simulink library "TYPEBP_MASTER_tmp"  (Simulink 8.6)
settings: Solver=ode45  StartTime=0.0  StopTime=10.0  RelTol=1e-3
undefined symbols (not defined in the file): TYPEC, TYPEC_MASTER
libraries: cdsEpicsOut x112, cdsFilt x79, cdsTP x59, cdsFiltCtrl x36, VIS_LIB x20, cdsEpicsIn x18, cdsMuxMatrix x14, STATE_BIO_MASTER x12, cdsEpicsBinIn x8, cdsFunctionCall x4, lockin x4, cdsEpicsStringIn x2
(part 12 of 13)

== system TYPEBP_MASTER_tmp/TYPEBPMASTER_TEST/SF/TEST ==
  GAS : cdsFilt/Subsystem  Tag=cdsFilt  Description=|
      | Purpose:                                                                                                                                                                                                                                  
      | Standard CDS IIR filter module.                                                                                                                                                                                                           
      |                                                                                                                                                                                                                                           
      | Operation:                                                                                                                                                                                                                                
      | Consists of 10 second order section IIR filters, plus a ramped gain stage. In FE code, also provides pre-defined test points and excitation channel inputs. The filter coefficients are defined in the LIGO system using the 'foton' tool.
      |                                                                                                                                                                                                                                           
      | Usage:                                                                                                                                                                                                                                    
      | Name the part with the desired filter module name.
      settings: AttributesFormatString=%<Tag>
  Ground1 : Ground
  Ground7 : Ground
  STATUS : cdsEpicsBinIn/Subsystem  Tag=cdsEpicsBinIn  Description=|
      | Purpose:                                                                            
      | Create an EPICS binary (0 or 1) input channel to the FE realtime controls.          
      |                                                                                     
      | Operation:                                                                          
      | Outputs value from an EPICS ai record. Value is binary input (bi Epics record type).
      |                                                                                     
      | Usage:                                                                              
      | Name the part with the desired EPICS channel name.
      settings: AttributesFormatString=%<Tag>
  F0_Out : Outport
  wires:
  GAS/1 -> F0_Out/1
  Ground1/1 -> GAS/1
  Ground7/1 -> STATUS/1

== system TYPEBP_MASTER_tmp/TYPEBPMASTER_TEST/TM/ADD ==
  ISC_L_In : Inport
  ISC_P_In : Inport  Port=2
  ISC_Y_In : Inport  Port=3
  TEST_L_In : Inport  Port=4
  TEST_P_In : Inport  Port=5
  TEST_Y_In : Inport  Port=6
  DAMP_L_In : Inport  Port=7
  DAMP_P_In : Inport  Port=8
  DAMP_Y_In : Inport  Port=9
  Ground{1..6} (6 alike) : Ground
  L : cdsFiltCtrl/IIR FM with control  Tag=cdsFiltCtrl  Description=|
      | cdsFiltCntrl is the standard IIR filter module (exactly the same as cdsFilt) but with added control data output 'Ctrl'. Filter module digital signal output appears on the first output, which is called 'Val'. 'Ctrl' output has a bit pattern encoding the state of filter's on/off switches (FM1 through FM10). The bit values are:
      |                                                                                                                                                                                                                                                                                                                                       
      | module 	hex	dec                                                                                                                                                                                                                                                                                                                       
      | -----------------------                                                                                                                                                                                                                                                                                                               
      | FM1	0x20                    32                                                                                                                                                                                                                                                                                                        
      | FM2	0x80                     128                                                                                                                                                                                                                                                                                                      
      | FM3	0x200                   512                                                                                                                                                                                                                                                                                                       
      | FM4	0x800                   2048                                                                                                                                                                                                                                                                                                      
      | FM5	0x2000                 8192                                                                                                                                                                                                                                                                                                       
      | FM6	0x8000                 32768                                                                                                                                                                                                                                                                                                      
      | FM7	0x20000                131072                                                                                                                                                                                                                                                                                                     
      | FM8	0x80000                 524288                                                                                                                                                                                                                                                                                                    
      | FM9	0x200000               2097152                                                                                                                                                                                                                                                                                                    
      | FM10	0x800000               8388608                                                                                                                                                                                                                                                                                                   
      |                                                                                                                                                                                                                                                                                                                                       
      | This bit data can be used to drive some other switches or it can be output using a binary I/O module.
      settings: AttributesFormatString=%<Tag>
  P : cdsFiltCtrl/IIR FM with control  Tag=cdsFiltCtrl  Description=|
      | cdsFiltCntrl is the standard IIR filter module (exactly the same as cdsFilt) but with added control data output 'Ctrl'. Filter module digital signal output appears on the first output, which is called 'Val'. 'Ctrl' output has a bit pattern encoding the state of filter's on/off switches (FM1 through FM10). The bit values are:
      |                                                                                                                                                                                                                                                                                                                                       
      | module 	hex	dec                                                                                                                                                                                                                                                                                                                       
      | -----------------------                                                                                                                                                                                                                                                                                                               
      | FM1	0x20                    32                                                                                                                                                                                                                                                                                                        
      | FM2	0x80                     128                                                                                                                                                                                                                                                                                                      
      | FM3	0x200                   512                                                                                                                                                                                                                                                                                                       
      | FM4	0x800                   2048                                                                                                                                                                                                                                                                                                      
      | FM5	0x2000                 8192                                                                                                                                                                                                                                                                                                       
      | FM6	0x8000                 32768                                                                                                                                                                                                                                                                                                      
      | FM7	0x20000                131072                                                                                                                                                                                                                                                                                                     
      | FM8	0x80000                 524288                                                                                                                                                                                                                                                                                                    
      | FM9	0x200000               2097152                                                                                                                                                                                                                                                                                                    
      | FM10	0x800000               8388608                                                                                                                                                                                                                                                                                                   
      |                                                                                                                                                                                                                                                                                                                                       
      | This bit data can be used to drive some other switches or it can be output using a binary I/O module.
      settings: AttributesFormatString=%<Tag>
  Sum : Sum  Inputs=+++
  Sum3 : Sum  Inputs=+++
  Sum4 : Sum  Inputs=+++
  Terminator1 : Terminator
  Terminator2 : Terminator
  Terminator3 : Terminator
  Y : cdsFiltCtrl/IIR FM with control  Tag=cdsFiltCtrl  Description=|
      | cdsFiltCntrl is the standard IIR filter module (exactly the same as cdsFilt) but with added control data output 'Ctrl'. Filter module digital signal output appears on the first output, which is called 'Val'. 'Ctrl' output has a bit pattern encoding the state of filter's on/off switches (FM1 through FM10). The bit values are:
      |                                                                                                                                                                                                                                                                                                                                       
      | module 	hex	dec                                                                                                                                                                                                                                                                                                                       
      | -----------------------                                                                                                                                                                                                                                                                                                               
      | FM1	0x20                    32                                                                                                                                                                                                                                                                                                        
      | FM2	0x80                     128                                                                                                                                                                                                                                                                                                      
      | FM3	0x200                   512                                                                                                                                                                                                                                                                                                       
      | FM4	0x800                   2048                                                                                                                                                                                                                                                                                                      
      | FM5	0x2000                 8192                                                                                                                                                                                                                                                                                                       
      | FM6	0x8000                 32768                                                                                                                                                                                                                                                                                                      
      | FM7	0x20000                131072                                                                                                                                                                                                                                                                                                     
      | FM8	0x80000                 524288                                                                                                                                                                                                                                                                                                    
      | FM9	0x200000               2097152                                                                                                                                                                                                                                                                                                    
      | FM10	0x800000               8388608                                                                                                                                                                                                                                                                                                   
      |                                                                                                                                                                                                                                                                                                                                       
      | This bit data can be used to drive some other switches or it can be output using a binary I/O module.
      settings: AttributesFormatString=%<Tag>
  LONG_Out : Outport
  PITCH_Out : Outport  Port=2
  YAW_Out : Outport  Port=3
  wires:
  DAMP_Y_In/1 -> Sum3/3
  DAMP_P_In/1 -> Sum4/3
  DAMP_L_In/1 -> Sum/3
  ISC_L_In/1 -> Sum/1
  TEST_L_In/1 -> Sum/2
  ISC_Y_In/1 -> Sum3/1
  TEST_Y_In/1 -> Sum3/2
  TEST_P_In/1 -> Sum4/2
  ISC_P_In/1 -> Sum4/1
  Sum/1 -> L/1
  Ground1/1 -> L/3
  Ground6/1 -> L/2
  L/1 -> LONG_Out/1
  Sum4/1 -> P/1
  Ground2/1 -> P/3
  Ground3/1 -> P/2
  P/1 -> PITCH_Out/1
  Sum3/1 -> Y/1
  Ground4/1 -> Y/3
  Ground5/1 -> Y/2
  Y/1 -> YAW_Out/1
  L/2 -> Terminator1/1
  P/2 -> Terminator2/1
  Y/2 -> Terminator3/1

== system TYPEBP_MASTER_tmp/TYPEBPMASTER_TEST/TM/ADDASC ==
  ISC_P_In : Inport
  ISC_Y_In : Inport  Port=2
  DITHER_P_In : Inport  Port=3
  DITHER_Y_In : Inport  Port=4
  Sum3 : Sum
  Sum4 : Sum
  PITCH_Out : Outport
  YAW_Out : Outport  Port=2
  wires:
  DITHER_Y_In/1 -> Sum3/2
  DITHER_P_In/1 -> Sum4/2
  Sum4/1 -> PITCH_Out/1
  ISC_Y_In/1 -> Sum3/1
  ISC_P_In/1 -> Sum4/1
  Sum3/1 -> YAW_Out/1

== system TYPEBP_MASTER_tmp/TYPEBPMASTER_TEST/TM/DRIVEALIGN ==
  note: This could/should be replaced by
      | the CDS_PART cdsFiltMuxMatrix,
      | but I'm not sure how that works
      | in MEDM land just yet
      | -- JSK Feb 2011
  LONG_In : Inport
  PITCH_In : Inport  Port=2
  YAW_In : Inport  Port=3
  L2L : cdsFilt/Subsystem  Tag=cdsFilt  Description=|
      | Purpose:                                                                                                                                                                                                                                  
      | Standard CDS IIR filter module.                                                                                                                                                                                                           
      |                                                                                                                                                                                                                                           
      | Operation:                                                                                                                                                                                                                                
      | Consists of 10 second order section IIR filters, plus a ramped gain stage. In FE code, also provides pre-defined test points and excitation channel inputs. The filter coefficients are defined in the LIGO system using the 'foton' tool.
      |                                                                                                                                                                                                                                           
      | Usage:                                                                                                                                                                                                                                    
      | Name the part with the desired filter module name.
      settings: AttributesFormatString=%<Tag>
  L2P : cdsFilt/Subsystem  Tag=cdsFilt  Description=|
      | Purpose:                                                                                                                                                                                                                                  
      | Standard CDS IIR filter module.                                                                                                                                                                                                           
      |                                                                                                                                                                                                                                           
      | Operation:                                                                                                                                                                                                                                
      | Consists of 10 second order section IIR filters, plus a ramped gain stage. In FE code, also provides pre-defined test points and excitation channel inputs. The filter coefficients are defined in the LIGO system using the 'foton' tool.
      |                                                                                                                                                                                                                                           
      | Usage:                                                                                                                                                                                                                                    
      | Name the part with the desired filter module name.
      settings: AttributesFormatString=%<Tag>
  L2Y : cdsFilt/Subsystem  Tag=cdsFilt  Description=|
      | Purpose:                                                                                                                                                                                                                                  
      | Standard CDS IIR filter module.                                                                                                                                                                                                           
      |                                                                                                                                                                                                                                           
      | Operation:                                                                                                                                                                                                                                
      | Consists of 10 second order section IIR filters, plus a ramped gain stage. In FE code, also provides pre-defined test points and excitation channel inputs. The filter coefficients are defined in the LIGO system using the 'foton' tool.
      |                                                                                                                                                                                                                                           
      | Usage:                                                                                                                                                                                                                                    
      | Name the part with the desired filter module name.
      settings: AttributesFormatString=%<Tag>
  L_IN : cdsTP/Subsystem  Tag=Test Point
      settings: AttributesFormatString=%<Tag>
  L_INMON : cdsEpicsOut/Subsystem  Tag=cdsEpicsOutput  Description=|
      | Purpose:                                          
      | Output a FE signal to an EPICS channel.           
      |                                                   
      | Operation:                                        
      | Takes input value and passes it to EPICS record.  
      |                                                   
      | Usage:                                            
      | Name the part with the desired EPICS rrecord name.
      settings: AttributesFormatString=%<Tag>
  L_OUT : cdsTP/Subsystem  Tag=Test Point
      settings: AttributesFormatString=%<Tag>
  L_OUTMON : cdsEpicsOut/Subsystem  Tag=cdsEpicsOutput  Description=|
      | Purpose:                                          
      | Output a FE signal to an EPICS channel.           
      |                                                   
      | Operation:                                        
      | Takes input value and passes it to EPICS record.  
      |                                                   
      | Usage:                                            
      | Name the part with the desired EPICS rrecord name.
      settings: AttributesFormatString=%<Tag>
  P2L : cdsFilt/Subsystem  Tag=cdsFilt  Description=|
      | Purpose:                                                                                                                                                                                                                                  
      | Standard CDS IIR filter module.                                                                                                                                                                                                           
      |                                                                                                                                                                                                                                           
      | Operation:                                                                                                                                                                                                                                
      | Consists of 10 second order section IIR filters, plus a ramped gain stage. In FE code, also provides pre-defined test points and excitation channel inputs. The filter coefficients are defined in the LIGO system using the 'foton' tool.
      |                                                                                                                                                                                                                                           
      | Usage:                                                                                                                                                                                                                                    
      | Name the part with the desired filter module name.
      settings: AttributesFormatString=%<Tag>
  P2P : cdsFilt/Subsystem  Tag=cdsFilt  Description=|
      | Purpose:                                                                                                                                                                                                                                  
      | Standard CDS IIR filter module.                                                                                                                                                                                                           
      |                                                                                                                                                                                                                                           
      | Operation:                                                                                                                                                                                                                                
      | Consists of 10 second order section IIR filters, plus a ramped gain stage. In FE code, also provides pre-defined test points and excitation channel inputs. The filter coefficients are defined in the LIGO system using the 'foton' tool.
      |                                                                                                                                                                                                                                           
      | Usage:                                                                                                                                                                                                                                    
      | Name the part with the desired filter module name.
      settings: AttributesFormatString=%<Tag>
  P2Y : cdsFilt/Subsystem  Tag=cdsFilt  Description=|
      | Purpose:                                                                                                                                                                                                                                  
      | Standard CDS IIR filter module.                                                                                                                                                                                                           
      |                                                                                                                                                                                                                                           
      | Operation:                                                                                                                                                                                                                                
      | Consists of 10 second order section IIR filters, plus a ramped gain stage. In FE code, also provides pre-defined test points and excitation channel inputs. The filter coefficients are defined in the LIGO system using the 'foton' tool.
      |                                                                                                                                                                                                                                           
      | Usage:                                                                                                                                                                                                                                    
      | Name the part with the desired filter module name.
      settings: AttributesFormatString=%<Tag>
  P_IN : cdsTP/Subsystem  Tag=Test Point
      settings: AttributesFormatString=%<Tag>
  P_INMON : cdsEpicsOut/Subsystem  Tag=cdsEpicsOutput  Description=|
      | Purpose:                                          
      | Output a FE signal to an EPICS channel.           
      |                                                   
      | Operation:                                        
      | Takes input value and passes it to EPICS record.  
      |                                                   
      | Usage:                                            
      | Name the part with the desired EPICS rrecord name.
      settings: AttributesFormatString=%<Tag>
  P_OUT : cdsTP/Subsystem  Tag=Test Point
      settings: AttributesFormatString=%<Tag>
  P_OUTMON : cdsEpicsOut/Subsystem  Tag=cdsEpicsOutput  Description=|
      | Purpose:                                          
      | Output a FE signal to an EPICS channel.           
      |                                                   
      | Operation:                                        
      | Takes input value and passes it to EPICS record.  
      |                                                   
      | Usage:                                            
      | Name the part with the desired EPICS rrecord name.
      settings: AttributesFormatString=%<Tag>
  Sum : Sum  Inputs=+++
  Sum1 : Sum  Inputs=+++
  Sum2 : Sum  Inputs=+++
  Y2L : cdsFilt/Subsystem  Tag=cdsFilt  Description=|
      | Purpose:                                                                                                                                                                                                                                  
      | Standard CDS IIR filter module.                                                                                                                                                                                                           
      |                                                                                                                                                                                                                                           
      | Operation:                                                                                                                                                                                                                                
      | Consists of 10 second order section IIR filters, plus a ramped gain stage. In FE code, also provides pre-defined test points and excitation channel inputs. The filter coefficients are defined in the LIGO system using the 'foton' tool.
      |                                                                                                                                                                                                                                           
      | Usage:                                                                                                                                                                                                                                    
      | Name the part with the desired filter module name.
      settings: AttributesFormatString=%<Tag>
  Y2P : cdsFilt/Subsystem  Tag=cdsFilt  Description=|
      | Purpose:                                                                                                                                                                                                                                  
      | Standard CDS IIR filter module.                                                                                                                                                                                                           
      |                                                                                                                                                                                                                                           
      | Operation:                                                                                                                                                                                                                                
      | Consists of 10 second order section IIR filters, plus a ramped gain stage. In FE code, also provides pre-defined test points and excitation channel inputs. The filter coefficients are defined in the LIGO system using the 'foton' tool.
      |                                                                                                                                                                                                                                           
      | Usage:                                                                                                                                                                                                                                    
      | Name the part with the desired filter module name.
      settings: AttributesFormatString=%<Tag>
  Y2Y : cdsFilt/Subsystem  Tag=cdsFilt  Description=|
      | Purpose:                                                                                                                                                                                                                                  
      | Standard CDS IIR filter module.                                                                                                                                                                                                           
      |                                                                                                                                                                                                                                           
      | Operation:                                                                                                                                                                                                                                
      | Consists of 10 second order section IIR filters, plus a ramped gain stage. In FE code, also provides pre-defined test points and excitation channel inputs. The filter coefficients are defined in the LIGO system using the 'foton' tool.
      |                                                                                                                                                                                                                                           
      | Usage:                                                                                                                                                                                                                                    
      | Name the part with the desired filter module name.
      settings: AttributesFormatString=%<Tag>
  Y_IN : cdsTP/Subsystem  Tag=Test Point
      settings: AttributesFormatString=%<Tag>
  Y_INMON : cdsEpicsOut/Subsystem  Tag=cdsEpicsOutput  Description=|
      | Purpose:                                          
      | Output a FE signal to an EPICS channel.           
      |                                                   
      | Operation:                                        
      | Takes input value and passes it to EPICS record.  
      |                                                   
      | Usage:                                            
      | Name the part with the desired EPICS rrecord name.
      settings: AttributesFormatString=%<Tag>
  Y_OUT : cdsTP/Subsystem  Tag=Test Point
      settings: AttributesFormatString=%<Tag>
  Y_OUTMON : cdsEpicsOut/Subsystem  Tag=cdsEpicsOutput  Description=|
      | Purpose:                                          
      | Output a FE signal to an EPICS channel.           
      |                                                   
      | Operation:                                        
      | Takes input value and passes it to EPICS record.  
      |                                                   
      | Usage:                                            
      | Name the part with the desired EPICS rrecord name.
      settings: AttributesFormatString=%<Tag>
  LONG_Out : Outport
  PITCH_Out : Outport  Port=2
  YAW_Out : Outport  Port=3
  wires:
  Y_OUTMON/1 -> YAW_Out/1
  P_OUTMON/1 -> PITCH_Out/1
  L_OUTMON/1 -> LONG_Out/1
  Y_INMON/1 -> Y_IN/1, Y2L/1, Y2Y/1, Y2P/1
  P_INMON/1 -> P_IN/1, P2L/1, P2Y/1, P2P/1
  L_INMON/1 -> L_IN/1, L2Y/1, L2P/1, L2L/1
  L2L/1 -> Sum/1
  P2L/1 -> Sum/2
  Y2L/1 -> Sum/3
  Y2P/1 -> Sum1/3
  P2P/1 -> Sum1/2
  L2P/1 -> Sum1/1
  Y2Y/1 -> Sum2/3
  P2Y/1 -> Sum2/2
  L2Y/1 -> Sum2/1
  Sum/1 -> L_OUT/1, L_OUTMON/1
  Sum1/1 -> P_OUT/1, P_OUTMON/1
  Sum2/1 -> Y_OUT/1, Y_OUTMON/1
  LONG_In/1 -> L_INMON/1
  PITCH_In/1 -> P_INMON/1
  YAW_In/1 -> Y_INMON/1

== system TYPEBP_MASTER_tmp/TYPEBPMASTER_TEST/TM/MASTER ==
  note: If second input (WDFLAG) is not equal to zero,
      | then pass out first argument (Constant 0 -- Block Output),
      | otherwise pass out third arguement (Constant 1 -- Pass Output)
  note: WDFLAG is 0 (zero) if OK,
      | Non-zero if BAD
  H1_In : Inport
  H2_In : Inport  Port=2
  H3_In : Inport  Port=3
  H4_In : Inport  Port=4
  MASTERSWITCH : Inport  Port=5
  WDFLAG : Inport  Port=6
  Add : Sum  Inputs=-+
  Constant1 : Constant
  OUT_H{1..4} (4 alike) : cdsTP/Subsystem  Tag=Test Point
      settings: AttributesFormatString=%<Tag>
  OUT_H1MON : cdsEpicsOut/Subsystem  Tag=cdsEpicsOutput  Description=|
      | Purpose:                                          
      | Output a FE signal to an EPICS channel.           
      |                                                   
      | Operation:                                        
      | Takes input value and passes it to EPICS record.  
      |                                                   
      | Usage:                                            
      | Name the part with the desired EPICS rrecord name.
      settings: AttributesFormatString=%<Tag>
  OUT_H2MON : cdsEpicsOut/Subsystem  Tag=cdsEpicsOutput  Description=|
      | Purpose:                                          
      | Output a FE signal to an EPICS channel.           
      |                                                   
      | Operation:                                        
      | Takes input value and passes it to EPICS record.  
      |                                                   
      | Usage:                                            
      | Name the part with the desired EPICS rrecord name.
      settings: AttributesFormatString=%<Tag>
  OUT_H3MON : cdsEpicsOut/Subsystem  Tag=cdsEpicsOutput  Description=|
      | Purpose:                                          
      | Output a FE signal to an EPICS channel.           
      |                                                   
      | Operation:                                        
      | Takes input value and passes it to EPICS record.  
      |                                                   
      | Usage:                                            
      | Name the part with the desired EPICS rrecord name.
      settings: AttributesFormatString=%<Tag>
  OUT_H4MON : cdsEpicsOut/Subsystem  Tag=cdsEpicsOutput  Description=|
      | Purpose:                                          
      | Output a FE signal to an EPICS channel.           
      |                                                   
      | Operation:                                        
      | Takes input value and passes it to EPICS record.  
      |                                                   
      | Usage:                                            
      | Name the part with the desired EPICS rrecord name.
      settings: AttributesFormatString=%<Tag>
  PWD_H{1..4} (4 alike) : cdsTP/Subsystem  Tag=Test Point
      settings: AttributesFormatString=%<Tag>
  PWD_H1MON : cdsEpicsOut/Subsystem  Tag=cdsEpicsOutput  Description=|
      | Purpose:                                          
      | Output a FE signal to an EPICS channel.           
      |                                                   
      | Operation:                                        
      | Takes input value and passes it to EPICS record.  
      |                                                   
      | Usage:                                            
      | Name the part with the desired EPICS rrecord name.
      settings: AttributesFormatString=%<Tag>
  PWD_H2MON : cdsEpicsOut/Subsystem  Tag=cdsEpicsOutput  Description=|
      | Purpose:                                          
      | Output a FE signal to an EPICS channel.           
      |                                                   
      | Operation:                                        
      | Takes input value and passes it to EPICS record.  
      |                                                   
      | Usage:                                            
      | Name the part with the desired EPICS rrecord name.
      settings: AttributesFormatString=%<Tag>
  PWD_H3MON : cdsEpicsOut/Subsystem  Tag=cdsEpicsOutput  Description=|
      | Purpose:                                          
      | Output a FE signal to an EPICS channel.           
      |                                                   
      | Operation:                                        
      | Takes input value and passes it to EPICS record.  
      |                                                   
      | Usage:                                            
      | Name the part with the desired EPICS rrecord name.
      settings: AttributesFormatString=%<Tag>
  PWD_H4MON : cdsEpicsOut/Subsystem  Tag=cdsEpicsOutput  Description=|
      | Purpose:                                          
      | Output a FE signal to an EPICS channel.           
      |                                                   
      | Operation:                                        
      | Takes input value and passes it to EPICS record.  
      |                                                   
      | Usage:                                            
      | Name the part with the desired EPICS rrecord name.
      settings: AttributesFormatString=%<Tag>
  P_MS_H{1..4} (4 alike) : Product  RndMeth=Zero
  P_WD_H{1..4} (4 alike) : Product  RndMeth=Zero
  SWITCHMON : cdsEpicsOut/Subsystem  Tag=cdsEpicsOutput  Description=|
      | Purpose:                                          
      | Output a FE signal to an EPICS channel.           
      |                                                   
      | Operation:                                        
      | Takes input value and passes it to EPICS record.  
      |                                                   
      | Usage:                                            
      | Name the part with the desired EPICS rrecord name.
      settings: AttributesFormatString=%<Tag>
  Terminator2 : Terminator
  H1_Out : Outport
  H2_Out : Outport  Port=2
  H3_Out : Outport  Port=3
  H4_Out : Outport  Port=4
  wires:
  Add/1 -> P_WD_H1/2, P_WD_H2/2, P_WD_H3/2, P_WD_H4/2
  PWD_H4MON/1 -> P_WD_H4/1
  PWD_H3MON/1 -> P_WD_H3/1
  PWD_H2MON/1 -> P_WD_H2/1
  PWD_H1MON/1 -> P_WD_H1/1
  H1_In/1 -> P_MS_H1/2
  H2_In/1 -> P_MS_H2/2
  H3_In/1 -> P_MS_H3/2
  H4_In/1 -> P_MS_H4/2
  MASTERSWITCH/1 -> P_MS_H4/1, P_MS_H3/1, P_MS_H2/1, P_MS_H1/1, SWITCHMON/1
  OUT_H2MON/1 -> H2_Out/1
  OUT_H1MON/1 -> H1_Out/1
  OUT_H3MON/1 -> H3_Out/1
  OUT_H4MON/1 -> H4_Out/1
  P_MS_H1/1 -> PWD_H1MON/1, PWD_H1/1
  P_MS_H2/1 -> PWD_H2MON/1, PWD_H2/1
  P_MS_H3/1 -> PWD_H3MON/1, PWD_H3/1
  P_MS_H4/1 -> PWD_H4MON/1, PWD_H4/1
  P_WD_H1/1 -> OUT_H1MON/1, OUT_H1/1
  P_WD_H2/1 -> OUT_H2MON/1, OUT_H2/1
  P_WD_H3/1 -> OUT_H3MON/1, OUT_H3/1
  P_WD_H4/1 -> OUT_H4MON/1, OUT_H4/1
  Constant1/1 -> Add/2
  WDFLAG/1 -> Add/1
  SWITCHMON/1 -> Terminator2/1
